simulink model "buoi2_DSB_SC"  (R2020b)
settings: Solver=VariableStepAuto  StartTime=0.0  StopTime=10.0  RelTol=1e-3
settings Model: Creator=htn  LastModifiedBy=htn

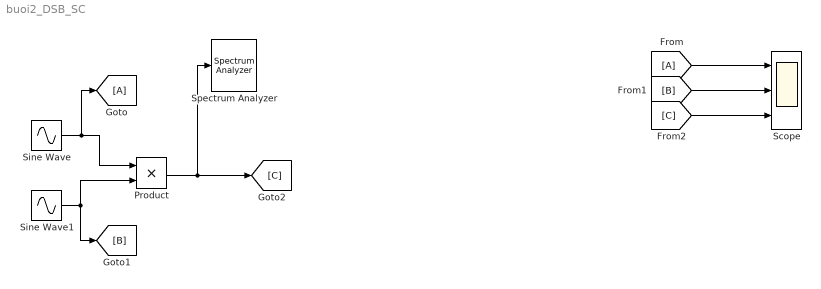
== system buoi2_DSB_SC ==
  Product : Product
  Scope : Scope  NumInputPorts=3
  Sine Wave : Sin  Frequency=2*pi*200  SampleTime=1/50000
  Sine Wave1 : Sin  Frequency=2*pi*5000  SampleTime=1/50000
  Spectrum Analyzer : SpectrumAnalyzer
  wires:
  Sine Wave/1 -> [A], Product/1
  Sine Wave1/1 -> [B], Product/2
  Product/1 -> Spectrum Analyzer/1, [C]
  [A] -> Scope/1
  [B] -> Scope/2
  [C] -> Scope/3
